simulink model "RL_UR3e_Pick_and_Place_Traj"  (R2024b)
settings: Solver=ode4  StartTime=0.0  StopTime=Tf  FixedStep=Ts_sim  RelTol=1e-3
values from neighbouring files (symbols this model uses):
  I_SCALE = 1 / I_max    (= 0.0104166666667)    [LQR_Gains.m]
  Ke = 0.0437    [LQR_Gains.m]
  Kt = 0.0437    [LQR_Gains.m]
  L = 0.001    [LQR_Gains.m]
  OMEGA_SCALE_J13 = 1 / pi    (= 0.318309886184)    [LQR_Gains.m]
  OMEGA_SCALE_J46 = 1 / (2*pi)    (= 0.159154943092)    [LQR_Gains.m]
  PICK = [-380, -170, 120]    [EvaluateAndAnalyzeAgents.m]    (also in Reward.m = PickTarget(:); TrainSACAgentForPickAndPlaceTraj.m; UR3eResetFcn.m; argetScheduler.m = Pick)
  PLACE = [-200,  -50, 300]    [EvaluateAndAnalyzeAgents.m]    (also in Reward.m = PlaceTarget(:); TrainSACAgentForPickAndPlaceTraj.m; UR3eResetFcn.m; argetScheduler.m = Place)
  R = 0.50    (= 0.5)    [LQR_Gains.m]
  Z_SCALE = Ts_sim    (= 0.005)    [LQR_Gains.m]
undefined symbols (not defined in the file or in its folder): b1, b2, b3, b4, b5, b6, InitTheta_1, InitTheta_2, InitTheta_3, InitTheta_4, InitTheta_5, InitTheta_6, J1, J2, J3, J4, J5, J6, K1, K2, K3, K4, K5, K6
libraries: rllib x1
(part 1 of 2)
settings Model: Creator=GigaByte Computers  LastModifiedBy=Acer
settings RTWCC: GPUComputeCapability=3.5

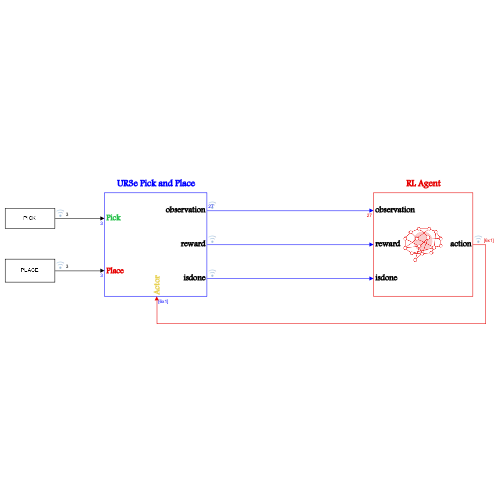
[thumbnail: Simulink's stored preview of the top-level diagram]
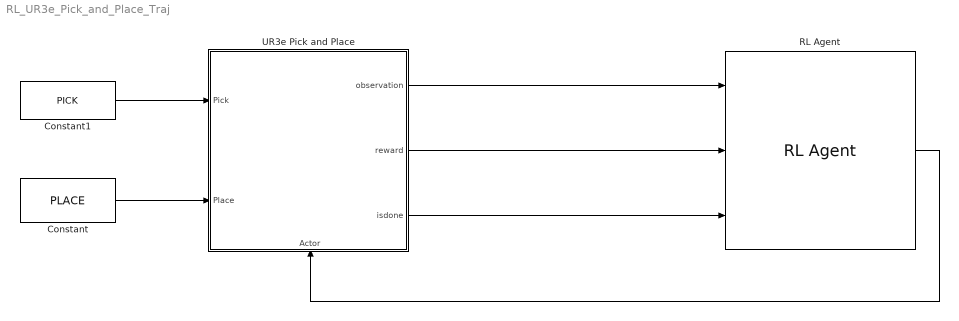
== system RL_UR3e_Pick_and_Place_Traj ==
  Constant : Constant  Value=PLACE
  Constant1 : Constant  Value=PICK
  RL Agent : rllib/RL Agent  Agent=agent  ExternalActionAsInput=off  ProvideLastAction=off  ProvideCumRwd=off  TreatAsDirectFeedthrough=on  UseStrictObservationDataTypes=off
  UR3e Pick and Place : Subsystem
      settings: PortSchema="{\"entries\":[{\"content\":{\"sides\":[{\"content\":{\"connectorIds\":[\"In1\",\"In2\"]},\"type\":\"ConnectorPlacement.EquallySpacedRectSide\",\"uuid\":\"13035aeb-c069-465b-bc28-233d93e7885c\"},{\"content\":{\"connectorIds\":[\"Out1\",\"Out2\",\"Out3\"],\"side\":\"RIGHT\"},\"type\":\"ConnectorPlacement.EquallySpacedRectSide\",\"uuid\":\"cbf2000c-b173-4779-ae30-0e5c1dcba60b\"},{\"content\":{\"connectorIds\":[\"In3\"],\"side\":\"TOP\"},\"type\":\"ConnectorPlacement.EquallySpacedRectSide\",\"uuid\":\"da0f4465-053c-4004-a8fa-0b8ae407464a\"}]},\"type\":\"ConnectorPlacement.EquallySpacedConnector\",\"uuid\":\"398c6cdf-546b-4a24-a522-29148214b593\"}],\"packageUris\":[\"http://schema.mathworks.com/mf0/Connector/R2020b\"],\"version\":\"1.0\"}"
  wires:
  UR3e Pick and Place/2(reward) -> RL Agent/2
  UR3e Pick and Place/1(isdone) -> RL Agent/3
  Constant/1 -> UR3e Pick and Place/1(Place)
  Constant1/1 -> UR3e Pick and Place/2(Pick)
  RL Agent/1 -> UR3e Pick and Place/3(Actor)
  UR3e Pick and Place/3(observation) -> RL Agent/1

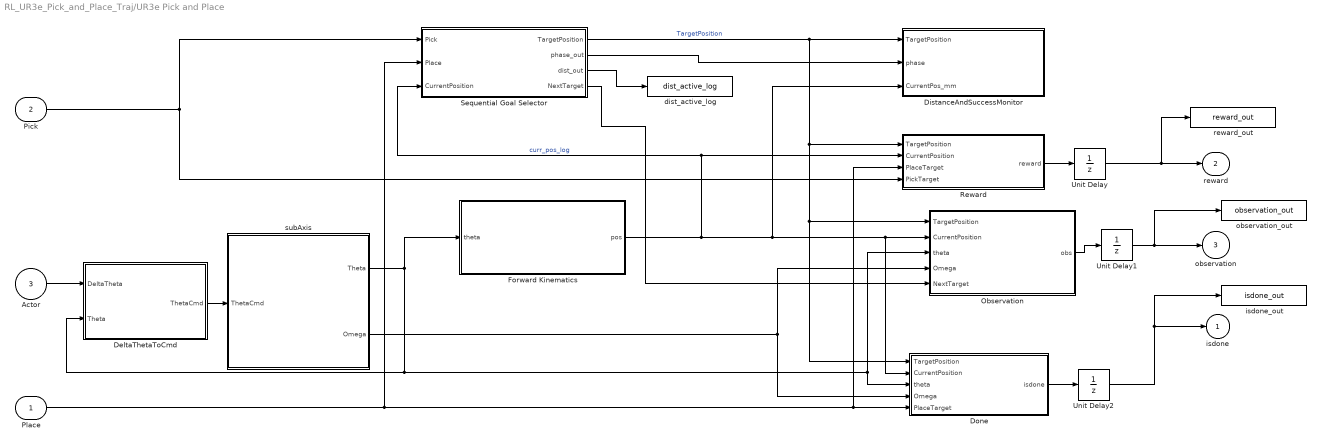
== system RL_UR3e_Pick_and_Place_Traj/UR3e Pick and Place ==
  Place : Inport
  Pick : Inport  Port=2
  Actor : Inport  Port=3
  DeltaThetaToCmd : MATLAB Function  TreatAsAtomicUnit=on
  DistanceAndSuccessMonitor : Subsystem
  Done : MATLAB Function
  Forward Kinematics : MATLAB Function
  Observation : MATLAB Function
  Reward : MATLAB Function
  Sequential Goal Selector : MATLAB Function  TreatAsAtomicUnit=on  SystemSampleTime=0.005
  Unit Delay : UnitDelay  SampleTime=-1  HasFrameUpgradeWarning=on
  Unit Delay1 : UnitDelay  SampleTime=-1  HasFrameUpgradeWarning=on
  Unit Delay2 : UnitDelay  InitialCondition=false  SampleTime=-1  HasFrameUpgradeWarning=on
  dist_active_log : ToWorkspace  VariableName=dist_active_log  SampleTime=-1
      settings: Save2DSignal=2-D array (concatenate along first dimension)
  isdone_out : ToWorkspace  VariableName=isdone_out  SampleTime=-1
      settings: Save2DSignal=2-D array (concatenate along first dimension)
  observation_out : ToWorkspace  VariableName=observation_out  SampleTime=-1
      settings: Save2DSignal=2-D array (concatenate along first dimension)
  reward_out : ToWorkspace  VariableName=reward_out  SampleTime=-1
      settings: Save2DSignal=2-D array (concatenate along first dimension)
  subAxis : Subsystem
  isdone : Outport
  reward : Outport  Port=2
  observation : Outport  Port=3
  wires:
  Reward/1(reward) -> Unit Delay/1
  Observation/1(obs) -> Unit Delay1/1
  Done/1(isdone) -> Unit Delay2/1
  Unit Delay/1 -> reward_out/1, reward/1
  Unit Delay1/1 -> observation_out/1, observation/1
  Unit Delay2/1 -> isdone_out/1, isdone/1
  subAxis/1(Theta) -> Forward Kinematics/1(theta), Observation/3(theta), Done/3(theta), DeltaThetaToCmd/2(Theta)
  subAxis/2(Omega) -> Observation/4(Omega), Done/4(Omega)
  Pick/1 -> Reward/4(PickTarget), Sequential Goal Selector/1(Pick)
  Place/1 -> Sequential Goal Selector/2(Place), Reward/3(PlaceTarget), Done/5(PlaceTarget)
  Sequential Goal Selector/1(TargetPosition) -> Reward/1(TargetPosition), Done/1(TargetPosition), Observation/1(TargetPosition), DistanceAndSuccessMonitor/1(TargetPosition)  "TargetPosition"
  Sequential Goal Selector/2(phase_out) -> DistanceAndSuccessMonitor/2(phase)
  Forward Kinematics/1(pos) -> Done/2(CurrentPosition), Observation/2(CurrentPosition), DistanceAndSuccessMonitor/3(CurrentPos_mm), Sequential Goal Selector/3(CurrentPosition), Reward/2(CurrentPosition)  "curr_pos_log"
  Sequential Goal Selector/3(dist_out) -> dist_active_log/1
  DeltaThetaToCmd/1(ThetaCmd) -> subAxis/1(ThetaCmd)
  Actor/1 -> DeltaThetaToCmd/1(DeltaTheta)
  Sequential Goal Selector/4(NextTarget) -> Observation/5(NextTarget)

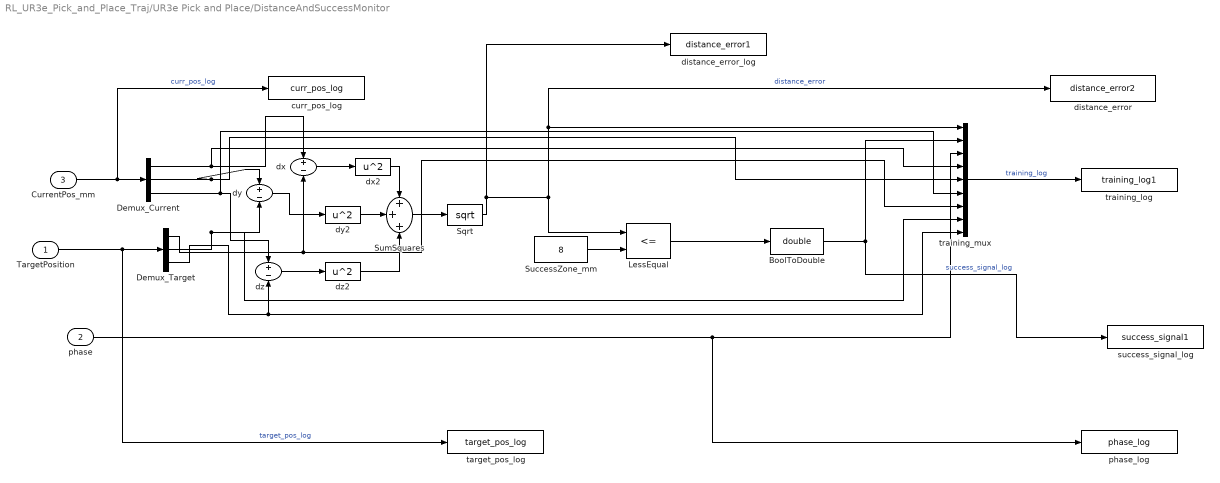
== system RL_UR3e_Pick_and_Place_Traj/UR3e Pick and Place/DistanceAndSuccessMonitor ==
  TargetPosition : Inport
  phase : Inport  Port=2
  CurrentPos_mm : Inport  Port=3
  BoolToDouble : DataTypeConversion  OutDataTypeStr=double  SaturateOnIntegerOverflow=off  RndMeth=Floor
  Demux_Current : Demux  Outputs=3
  Demux_Target : Demux  Outputs=3
  LessEqual : RelationalOperator  Operator=<=  OutDataTypeStr=boolean  RndMeth=Simplest  InputSameDT=off
  Sqrt : Math  Operator=sqrt
  SuccessZone_mm : Constant  Value=8
  SumSquares : Sum  Inputs=+++
  curr_pos_log : ToWorkspace  VariableName=curr_pos_log  SampleTime=-1
      settings: Save2DSignal=2-D array (concatenate along first dimension)
  distance_error : ToWorkspace  VariableName=distance_error2  SampleTime=-1
      settings: Save2DSignal=2-D array (concatenate along first dimension)
  distance_error_log : ToWorkspace  VariableName=distance_error1  SampleTime=-1
      settings: Save2DSignal=2-D array (concatenate along first dimension)
  dx : Sum  Inputs=+-
  dx2 : Math  Operator=square
  dy : Sum  Inputs=+-
  dy2 : Math  Operator=square
  dz : Sum  Inputs=+-
  dz2 : Math  Operator=square
  phase_log : ToWorkspace  VariableName=phase_log  SampleTime=-1
      settings: Save2DSignal=2-D array (concatenate along first dimension)
  success_signal_log : ToWorkspace  VariableName=success_signal1  SampleTime=-1
      settings: Save2DSignal=2-D array (concatenate along first dimension)
  target_pos_log : ToWorkspace  VariableName=target_pos_log  SampleTime=-1
      settings: Save2DSignal=2-D array (concatenate along first dimension)
  training_log : ToWorkspace  VariableName=training_log1  SampleTime=-1
      settings: Save2DSignal=2-D array (concatenate along first dimension)
  training_mux : Mux  Inputs=9
  wires:
  training_mux/1 -> training_log/1  "training_log"
  Demux_Target/1 -> dx/2, training_mux/7
  Demux_Target/3 -> dz/2, training_mux/9
  Demux_Current/2 -> dy/1, training_mux/5
  phase/1 -> phase_log/1, training_mux/3
  SuccessZone_mm/1 -> LessEqual/2
  Demux_Current/3 -> dz/1, training_mux/6
  dx2/1 -> SumSquares/1
  dy2/1 -> SumSquares/2
  dz2/1 -> SumSquares/3
  Sqrt/1 -> distance_error/1, training_mux/1, LessEqual/1, distance_error_log/1  "distance_error"
  SumSquares/1 -> Sqrt/1
  Demux_Target/2 -> dy/2, training_mux/8
  BoolToDouble/1 -> success_signal_log/1, training_mux/2  "success_signal_log"
  dy/1 -> dy2/1
  dz/1 -> dz2/1
  dx/1 -> dx2/1
  Demux_Current/1 -> dx/1, training_mux/4
  LessEqual/1 -> BoolToDouble/1
  TargetPosition/1 -> Demux_Target/1, target_pos_log/1  "target_pos_log"
  CurrentPos_mm/1 -> curr_pos_log/1, Demux_Current/1  "curr_pos_log"

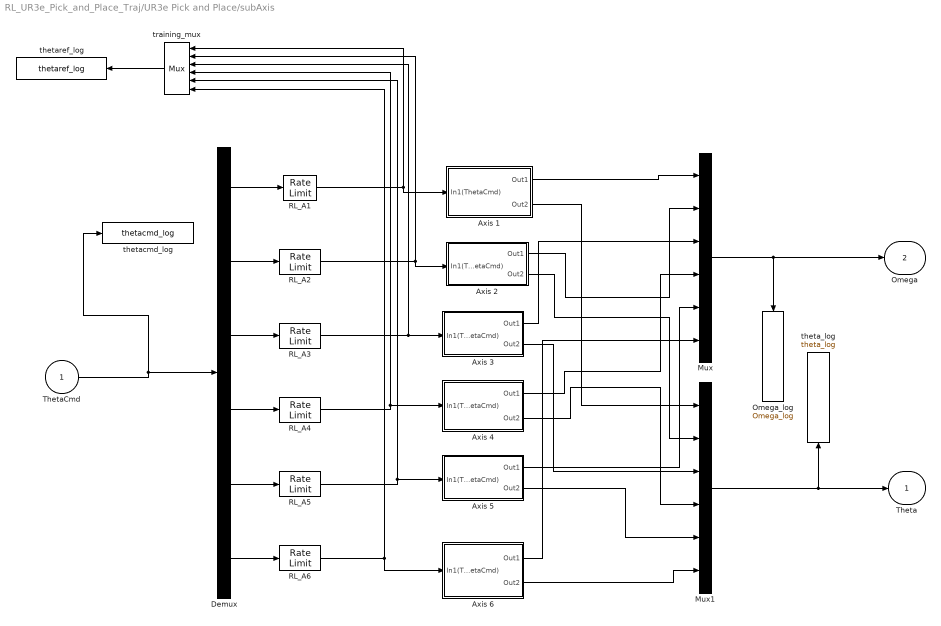
== system RL_UR3e_Pick_and_Place_Traj/UR3e Pick and Place/subAxis ==
  ThetaCmd : Inport
  Axis 1 : Subsystem
  Axis 2 : Subsystem
  Axis 3 : Subsystem
  Axis 4 : Subsystem
  Axis 5 : Subsystem
  Axis 6 : Subsystem
  Demux : Demux  Outputs=6
  Mux : Mux  Inputs=6
  Mux1 : Mux  Inputs=6
  Omega_log : ToWorkspace  VariableName=Omega_log  SampleTime=-1
      settings: Save2DSignal=2-D array (concatenate along first dimension)
  RL_A1 : RateLimiter  RisingSlewLimit=1*pi  FallingSlewLimit=-1*pi  SampleTimeMode=inherited
  RL_A2 : RateLimiter  RisingSlewLimit=1*pi  FallingSlewLimit=-1*pi  SampleTimeMode=inherited
  RL_A3 : RateLimiter  RisingSlewLimit=1*pi  FallingSlewLimit=-1*pi  SampleTimeMode=inherited
  RL_A4 : RateLimiter  RisingSlewLimit=2*pi  FallingSlewLimit=-2*pi  SampleTimeMode=inherited
  RL_A5 : RateLimiter  RisingSlewLimit=2*pi  FallingSlewLimit=-2*pi  SampleTimeMode=inherited
  RL_A6 : RateLimiter  RisingSlewLimit=2*pi  FallingSlewLimit=-2*pi  SampleTimeMode=inherited
  theta_log : ToWorkspace  VariableName=theta_log  SampleTime=-1
      settings: Save2DSignal=2-D array (concatenate along first dimension)
  thetacmd_log : ToWorkspace  VariableName=thetacmd_log  SampleTime=-1
      settings: Save2DSignal=2-D array (concatenate along first dimension)
  thetaref_log : ToWorkspace  VariableName=thetaref_log  SampleTime=-1
      settings: Save2DSignal=2-D array (concatenate along first dimension)
  training_mux : Mux  Inputs=6
  Theta : Outport
  Omega : Outport  Port=2
  wires:
  Demux/5 -> RL_A5/1
  Axis 5/1(Out1) -> Mux/5
  Axis 6/1(Out1) -> Mux/6
  Axis 2/2(Out2) -> Mux1/2
  Axis 3/2(Out2) -> Mux1/3
  Axis 5/2(Out2) -> Mux1/5
  Axis 2/1(Out1) -> Mux/2
  Demux/2 -> RL_A2/1
  Demux/3 -> RL_A3/1
  Axis 4/2(Out2) -> Mux1/4
  Demux/1 -> RL_A1/1
  Axis 1/1(Out1) -> Mux/1
  Axis 1/2(Out2) -> Mux1/1
  Axis 4/1(Out1) -> Mux/4
  Demux/4 -> RL_A4/1
  Axis 6/2(Out2) -> Mux1/6
  Demux/6 -> RL_A6/1
  Axis 3/1(Out1) -> Mux/3
  Mux1/1 -> Theta/1, theta_log/1
  ThetaCmd/1 -> Demux/1, thetacmd_log/1
  Mux/1 -> Omega_log/1, Omega/1
  RL_A1/1 -> Axis 1/1(In1(ThetaCmd)), training_mux/1
  RL_A6/1 -> Axis 6/1(In1(ThetaCmd)), training_mux/6
  RL_A2/1 -> Axis 2/1(In1(ThetaCmd)), training_mux/2
  RL_A3/1 -> training_mux/3, Axis 3/1(In1(ThetaCmd))
  RL_A4/1 -> Axis 4/1(In1(ThetaCmd)), training_mux/4
  RL_A5/1 -> Axis 5/1(In1(ThetaCmd)), training_mux/5
  training_mux/1 -> thetaref_log/1

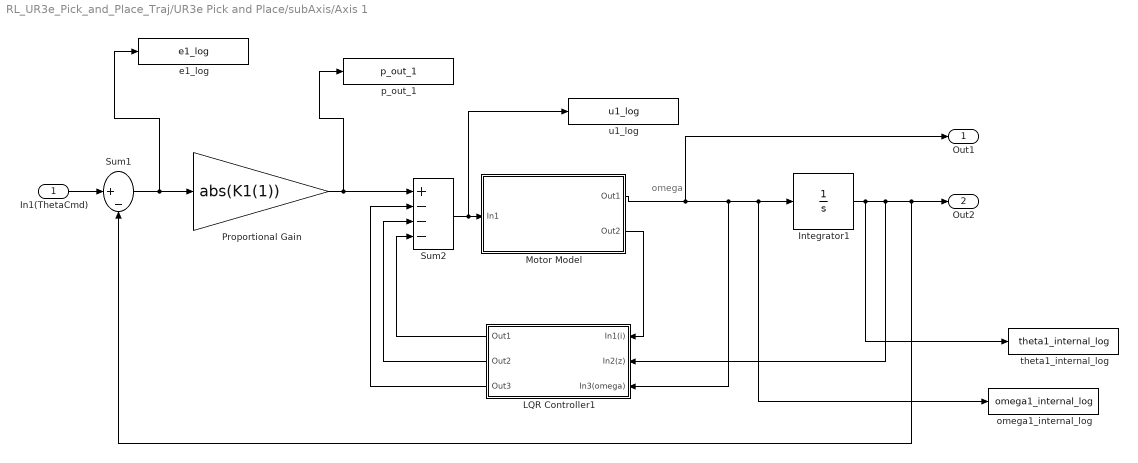
== system RL_UR3e_Pick_and_Place_Traj/UR3e Pick and Place/subAxis/Axis 1 ==
  note: omega
  In1(ThetaCmd) : Inport
  Integrator1 : Integrator  InitialCondition=InitTheta_1
  LQR Controller1 : Subsystem
  Motor Model : Subsystem
  Proportional Gain : Gain  Gain=abs(K1(1))
  Sum1 : Sum  Inputs=|+-
  Sum2 : Sum  Inputs=+---
  e1_log : ToWorkspace  VariableName=e1_log  SampleTime=-1
      settings: Save2DSignal=2-D array (concatenate along first dimension)
  omega1_internal_log : ToWorkspace  VariableName=omega1_internal_log  SampleTime=-1
      settings: Save2DSignal=2-D array (concatenate along first dimension)
  p_out_1 : ToWorkspace  VariableName=p_out_1  SampleTime=-1
      settings: Save2DSignal=2-D array (concatenate along first dimension)
  theta1_internal_log : ToWorkspace  VariableName=theta1_internal_log  SampleTime=-1
      settings: Save2DSignal=2-D array (concatenate along first dimension)
  u1_log : ToWorkspace  VariableName=u1_log  SampleTime=-1
      settings: Save2DSignal=2-D array (concatenate along first dimension)
  Out1 : Outport
  Out2 : Outport  Port=2
  wires:
  Sum2/1 -> u1_log/1, Motor Model/1(In1)
  Motor Model/1(Out1) -> Out1/1, LQR Controller1/3(In3(omega)), omega1_internal_log/1, Integrator1/1
  Sum1/1 -> e1_log/1, Proportional Gain/1
  Proportional Gain/1 -> p_out_1/1, Sum2/1
  In1(ThetaCmd)/1 -> Sum1/1
  LQR Controller1/1(Out1) -> Sum2/4
  LQR Controller1/2(Out2) -> Sum2/3
  LQR Controller1/3(Out3) -> Sum2/2
  Integrator1/1 -> theta1_internal_log/1, LQR Controller1/2("In2(z) "), Sum1/2, Out2/1
  Motor Model/2(Out2) -> LQR Controller1/1("In1(i) ")

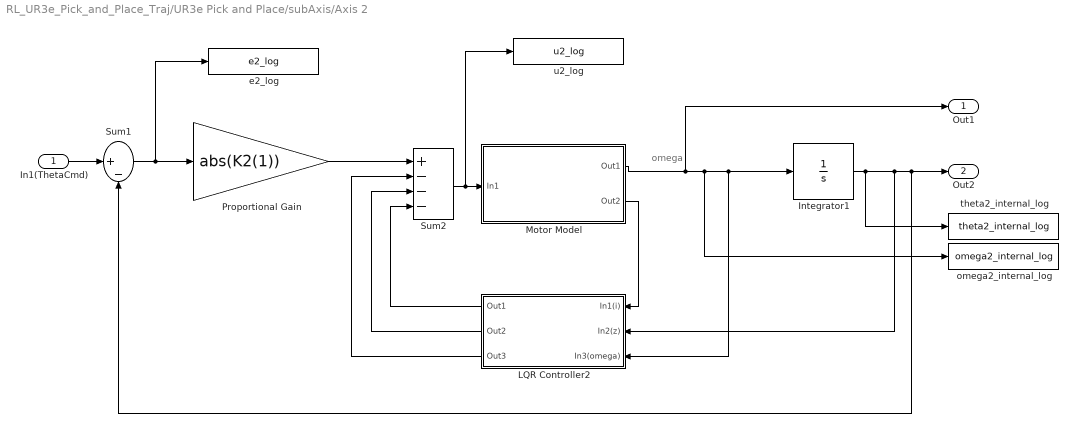
== system RL_UR3e_Pick_and_Place_Traj/UR3e Pick and Place/subAxis/Axis 2 ==
  note: omega
  In1(ThetaCmd) : Inport
  Integrator1 : Integrator  InitialCondition=InitTheta_2
  LQR Controller2 : Subsystem
  Motor Model : Subsystem
  Proportional Gain : Gain  Gain=abs(K2(1))
  Sum1 : Sum  Inputs=|+-
  Sum2 : Sum  Inputs=+---
  e2_log : ToWorkspace  VariableName=e2_log  SampleTime=-1
      settings: Save2DSignal=2-D array (concatenate along first dimension)
  omega2_internal_log : ToWorkspace  VariableName=omega2_internal_log  SampleTime=-1
      settings: Save2DSignal=2-D array (concatenate along first dimension)
  theta2_internal_log : ToWorkspace  VariableName=theta2_internal_log  SampleTime=-1
      settings: Save2DSignal=2-D array (concatenate along first dimension)
  u2_log : ToWorkspace  VariableName=u2_log  SampleTime=-1
      settings: Save2DSignal=2-D array (concatenate along first dimension)
  Out1 : Outport
  Out2 : Outport  Port=2
  wires:
  Proportional Gain/1 -> Sum2/1
  Motor Model/1(Out1) -> Out1/1, omega2_internal_log/1, LQR Controller2/3(In3(omega)), Integrator1/1
  LQR Controller2/2(Out2) -> Sum2/3
  Motor Model/2(Out2) -> LQR Controller2/1("In1(i) ")
  In1(ThetaCmd)/1 -> Sum1/1
  LQR Controller2/3(Out3) -> Sum2/2
  LQR Controller2/1(Out1) -> Sum2/4
  Sum1/1 -> e2_log/1, Proportional Gain/1
  Integrator1/1 -> theta2_internal_log/1, LQR Controller2/2("In2(z) "), Sum1/2, Out2/1
  Sum2/1 -> u2_log/1, Motor Model/1(In1)

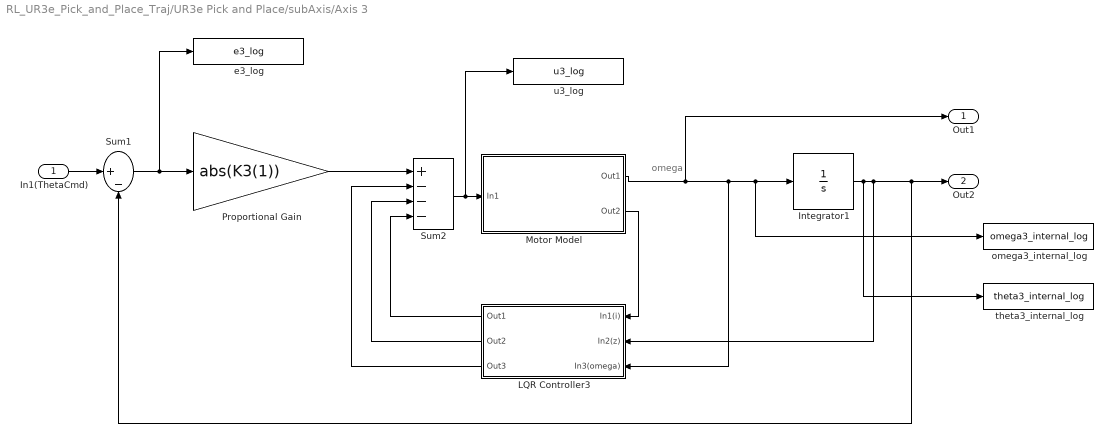
== system RL_UR3e_Pick_and_Place_Traj/UR3e Pick and Place/subAxis/Axis 3 ==
  note: omega
  In1(ThetaCmd) : Inport
  Integrator1 : Integrator  InitialCondition=InitTheta_3
  LQR Controller3 : Subsystem
  Motor Model : Subsystem
  Proportional Gain : Gain  Gain=abs(K3(1))
  Sum1 : Sum  Inputs=|+-
  Sum2 : Sum  Inputs=+---
  e3_log : ToWorkspace  VariableName=e3_log  SampleTime=-1
      settings: Save2DSignal=2-D array (concatenate along first dimension)
  omega3_internal_log : ToWorkspace  VariableName=omega3_internal_log  SampleTime=-1
      settings: Save2DSignal=2-D array (concatenate along first dimension)
  theta3_internal_log : ToWorkspace  VariableName=theta3_internal_log  SampleTime=-1
      settings: Save2DSignal=2-D array (concatenate along first dimension)
  u3_log : ToWorkspace  VariableName=u3_log  SampleTime=-1
      settings: Save2DSignal=2-D array (concatenate along first dimension)
  Out1 : Outport
  Out2 : Outport  Port=2
  wires:
  Sum2/1 -> u3_log/1, Motor Model/1(In1)
  Integrator1/1 -> theta3_internal_log/1, LQR Controller3/2("In2(z) "), Sum1/2, Out2/1
  Sum1/1 -> e3_log/1, Proportional Gain/1
  LQR Controller3/3(Out3) -> Sum2/2
  LQR Controller3/1(Out1) -> Sum2/4
  In1(ThetaCmd)/1 -> Sum1/1
  Motor Model/2(Out2) -> LQR Controller3/1("In1(i) ")
  Motor Model/1(Out1) -> Out1/1, omega3_internal_log/1, Integrator1/1, LQR Controller3/3(In3(omega))
  Proportional Gain/1 -> Sum2/1
  LQR Controller3/2(Out2) -> Sum2/3

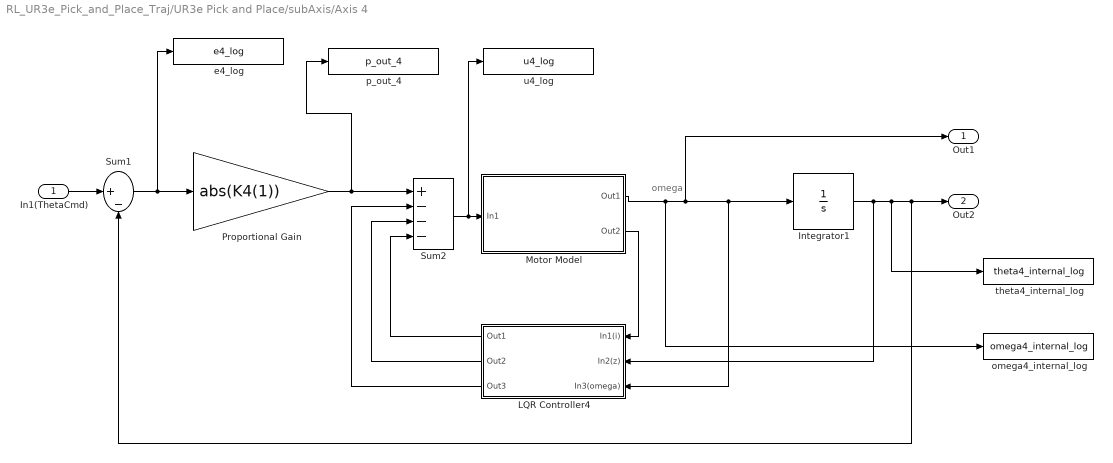
== system RL_UR3e_Pick_and_Place_Traj/UR3e Pick and Place/subAxis/Axis 4 ==
  note: omega
  In1(ThetaCmd) : Inport
  Integrator1 : Integrator  InitialCondition=InitTheta_4
  LQR Controller4 : Subsystem
  Motor Model : Subsystem
  Proportional Gain : Gain  Gain=abs(K4(1))
  Sum1 : Sum  Inputs=|+-
  Sum2 : Sum  Inputs=+---
  e4_log : ToWorkspace  VariableName=e4_log  SampleTime=-1
      settings: Save2DSignal=2-D array (concatenate along first dimension)
  omega4_internal_log : ToWorkspace  VariableName=omega4_internal_log  SampleTime=-1
      settings: Save2DSignal=2-D array (concatenate along first dimension)
  p_out_4 : ToWorkspace  VariableName=p_out_4  SampleTime=-1
      settings: Save2DSignal=2-D array (concatenate along first dimension)
  theta4_internal_log : ToWorkspace  VariableName=theta4_internal_log  SampleTime=-1
      settings: Save2DSignal=2-D array (concatenate along first dimension)
  u4_log : ToWorkspace  VariableName=u4_log  SampleTime=-1
      settings: Save2DSignal=2-D array (concatenate along first dimension)
  Out1 : Outport
  Out2 : Outport  Port=2
  wires:
  LQR Controller4/2(Out2) -> Sum2/3
  Proportional Gain/1 -> p_out_4/1, Sum2/1
  LQR Controller4/3(Out3) -> Sum2/2
  Sum1/1 -> e4_log/1, Proportional Gain/1
  Integrator1/1 -> LQR Controller4/2("In2(z) "), theta4_internal_log/1, Sum1/2, Out2/1
  Motor Model/1(Out1) -> omega4_internal_log/1, Out1/1, LQR Controller4/3(In3(omega)), Integrator1/1
  Motor Model/2(Out2) -> LQR Controller4/1("In1(i) ")
  LQR Controller4/1(Out1) -> Sum2/4
  In1(ThetaCmd)/1 -> Sum1/1
  Sum2/1 -> u4_log/1, Motor Model/1(In1)

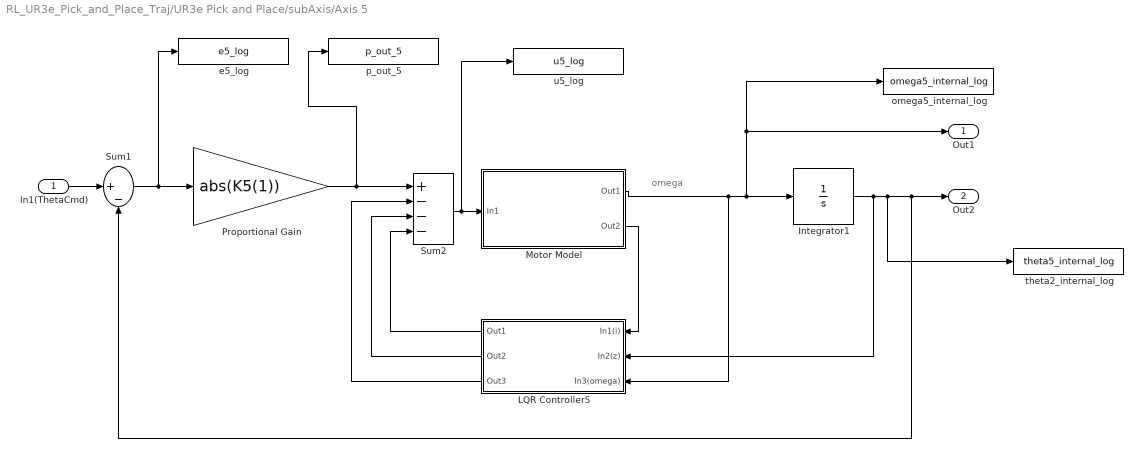
== system RL_UR3e_Pick_and_Place_Traj/UR3e Pick and Place/subAxis/Axis 5 ==
  note: omega
  In1(ThetaCmd) : Inport
  Integrator1 : Integrator  InitialCondition=InitTheta_5
  LQR Controller5 : Subsystem
  Motor Model : Subsystem
  Proportional Gain : Gain  Gain=abs(K5(1))
  Sum1 : Sum  Inputs=|+-
  Sum2 : Sum  Inputs=+---
  e5_log : ToWorkspace  VariableName=e5_log  SampleTime=-1
      settings: Save2DSignal=2-D array (concatenate along first dimension)
  omega5_internal_log : ToWorkspace  VariableName=omega5_internal_log  SampleTime=-1
      settings: Save2DSignal=2-D array (concatenate along first dimension)
  p_out_5 : ToWorkspace  VariableName=p_out_5  SampleTime=-1
      settings: Save2DSignal=2-D array (concatenate along first dimension)
  theta2_internal_log : ToWorkspace  VariableName=theta5_internal_log  SampleTime=-1
      settings: Save2DSignal=2-D array (concatenate along first dimension)
  u5_log : ToWorkspace  VariableName=u5_log  SampleTime=-1
      settings: Save2DSignal=2-D array (concatenate along first dimension)
  Out1 : Outport
  Out2 : Outport  Port=2
  wires:
  Proportional Gain/1 -> p_out_5/1, Sum2/1
  LQR Controller5/2(Out2) -> Sum2/3
  Sum2/1 -> u5_log/1, Motor Model/1(In1)
  Motor Model/2(Out2) -> LQR Controller5/1("In1(i) ")
  LQR Controller5/1(Out1) -> Sum2/4
  Motor Model/1(Out1) -> omega5_internal_log/1, Out1/1, Integrator1/1, LQR Controller5/3(In3(omega))
  In1(ThetaCmd)/1 -> Sum1/1
  Sum1/1 -> e5_log/1, Proportional Gain/1
  Integrator1/1 -> LQR Controller5/2("In2(z) "), theta2_internal_log/1, Sum1/2, Out2/1
  LQR Controller5/3(Out3) -> Sum2/2

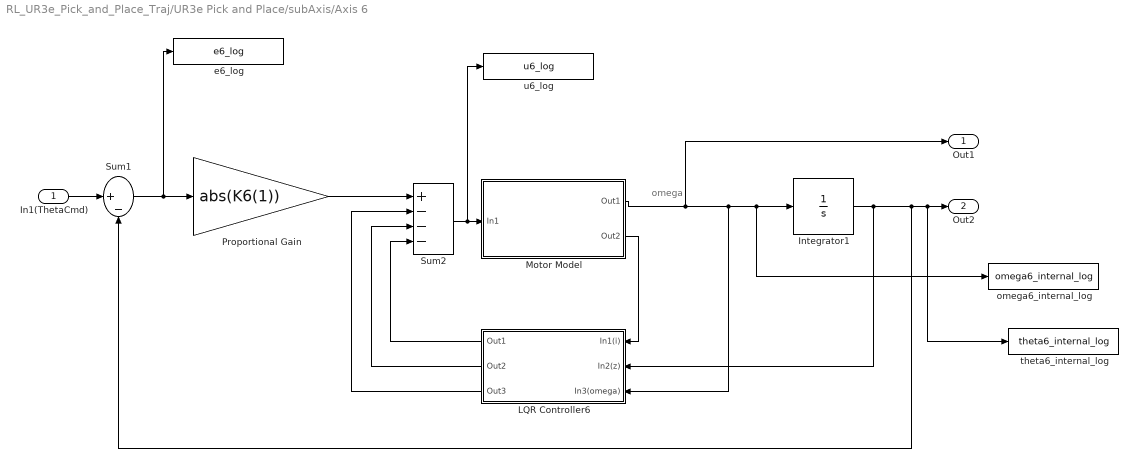
== system RL_UR3e_Pick_and_Place_Traj/UR3e Pick and Place/subAxis/Axis 6 ==
  note: omega
  In1(ThetaCmd) : Inport
  Integrator1 : Integrator  InitialCondition=InitTheta_6
  LQR Controller6 : Subsystem
  Motor Model : Subsystem
  Proportional Gain : Gain  Gain=abs(K6(1))
  Sum1 : Sum  Inputs=|+-
  Sum2 : Sum  Inputs=+---
  e6_log : ToWorkspace  VariableName=e6_log  SampleTime=-1
      settings: Save2DSignal=2-D array (concatenate along first dimension)
  omega6_internal_log : ToWorkspace  VariableName=omega6_internal_log  SampleTime=-1
      settings: Save2DSignal=2-D array (concatenate along first dimension)
  theta6_internal_log : ToWorkspace  VariableName=theta6_internal_log  SampleTime=-1
      settings: Save2DSignal=2-D array (concatenate along first dimension)
  u6_log : ToWorkspace  VariableName=u6_log  SampleTime=-1
      settings: Save2DSignal=2-D array (concatenate along first dimension)
  Out1 : Outport
  Out2 : Outport  Port=2
  wires:
  LQR Controller6/1(Out1) -> Sum2/4
  LQR Controller6/2(Out2) -> Sum2/3
  Motor Model/2(Out2) -> LQR Controller6/1("In1(i) ")
  Proportional Gain/1 -> Sum2/1
  Integrator1/1 -> LQR Controller6/2("In2(z) "), Sum1/2, theta6_internal_log/1, Out2/1
  Sum2/1 -> u6_log/1, Motor Model/1(In1)
  LQR Controller6/3(Out3) -> Sum2/2
  Motor Model/1(Out1) -> Out1/1, LQR Controller6/3(In3(omega)), omega6_internal_log/1, Integrator1/1
  Sum1/1 -> e6_log/1, Proportional Gain/1
  In1(ThetaCmd)/1 -> Sum1/1

== system RL_UR3e_Pick_and_Place_Traj/UR3e Pick and Place/subAxis/Axis 1/LQR Controller1 ==
  "In1(i) " : Inport
  "In2(z) " : Inport  Port=2
  In3(omega) : Inport  Port=3
  Gain omega : Gain  Gain=K1(3)*OMEGA_SCALE_J13
  Gain_i : Gain  Gain=K1(4)*I_SCALE
  Gain_z : Gain  Gain=K1(2)*Z_SCALE
  Out1 : Outport
  Out2 : Outport  Port=2
  Out3 : Outport  Port=3
  wires:
  "In2(z) "/1 -> Gain_z/1
  Gain_i/1 -> Out1/1
  "In1(i) "/1 -> Gain_i/1
  Gain omega/1 -> Out3/1
  Gain_z/1 -> Out2/1
  In3(omega)/1 -> Gain omega/1

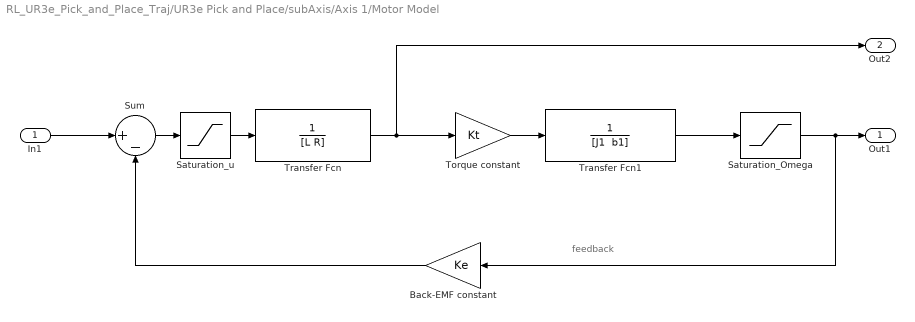
== system RL_UR3e_Pick_and_Place_Traj/UR3e Pick and Place/subAxis/Axis 1/Motor Model ==
  note: feedback
  In1 : Inport
  Back-EMF constant : Gain  Gain=Ke
  Saturation_Omega : Saturate  UpperLimit=1*pi  LowerLimit=-1*pi
  Saturation_u : Saturate  UpperLimit=48  LowerLimit=-48
  Sum : Sum  Inputs=|+-
  Torque constant : Gain  Gain=Kt
  Transfer Fcn : TransferFcn  Denominator=[L R]
  Transfer Fcn1 : TransferFcn  Denominator="[J1  b1]"
  Out1 : Outport
  Out2 : Outport  Port=2
  wires:
  In1/1 -> Sum/1
  Transfer Fcn/1 -> Torque constant/1, Out2/1
  Back-EMF constant/1 -> Sum/2
  Transfer Fcn1/1 -> Saturation_Omega/1
  Torque constant/1 -> Transfer Fcn1/1
  Sum/1 -> Saturation_u/1
  Saturation_u/1 -> Transfer Fcn/1
  Saturation_Omega/1 -> Back-EMF constant/1, Out1/1

== system RL_UR3e_Pick_and_Place_Traj/UR3e Pick and Place/subAxis/Axis 2/LQR Controller2 ==
  "In1(i) " : Inport
  "In2(z) " : Inport  Port=2
  In3(omega) : Inport  Port=3
  Gain omega : Gain  Gain=K2(3)*OMEGA_SCALE_J13
  Gain_i : Gain  Gain=K2(4)*I_SCALE
  Gain_z : Gain  Gain=K2(2)*Z_SCALE
  Out1 : Outport
  Out2 : Outport  Port=2
  Out3 : Outport  Port=3
  wires:
  "In2(z) "/1 -> Gain_z/1
  Gain_i/1 -> Out1/1
  "In1(i) "/1 -> Gain_i/1
  Gain omega/1 -> Out3/1
  Gain_z/1 -> Out2/1
  In3(omega)/1 -> Gain omega/1

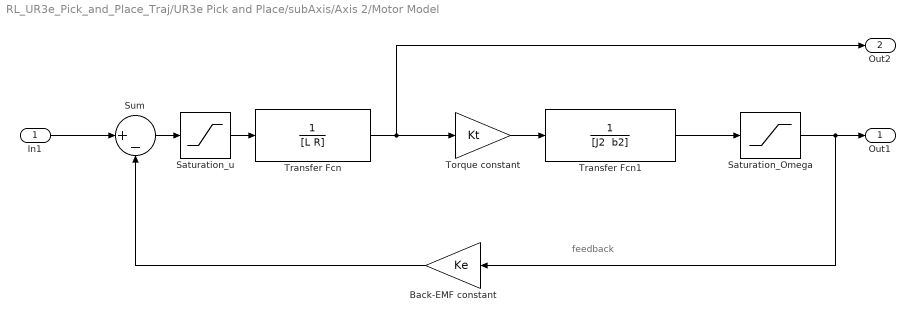
== system RL_UR3e_Pick_and_Place_Traj/UR3e Pick and Place/subAxis/Axis 2/Motor Model ==
  note: feedback
  In1 : Inport
  Back-EMF constant : Gain  Gain=Ke
  Saturation_Omega : Saturate  UpperLimit=1*pi  LowerLimit=-1*pi
  Saturation_u : Saturate  UpperLimit=48  LowerLimit=-48
  Sum : Sum  Inputs=|+-
  Torque constant : Gain  Gain=Kt
  Transfer Fcn : TransferFcn  Denominator=[L R]
  Transfer Fcn1 : TransferFcn  Denominator="[J2  b2]"
  Out1 : Outport
  Out2 : Outport  Port=2
  wires:
  In1/1 -> Sum/1
  Transfer Fcn/1 -> Torque constant/1, Out2/1
  Back-EMF constant/1 -> Sum/2
  Transfer Fcn1/1 -> Saturation_Omega/1
  Torque constant/1 -> Transfer Fcn1/1
  Sum/1 -> Saturation_u/1
  Saturation_u/1 -> Transfer Fcn/1
  Saturation_Omega/1 -> Back-EMF constant/1, Out1/1

== system RL_UR3e_Pick_and_Place_Traj/UR3e Pick and Place/subAxis/Axis 3/LQR Controller3 ==
  "In1(i) " : Inport
  "In2(z) " : Inport  Port=2
  In3(omega) : Inport  Port=3
  Gain omega : Gain  Gain=K3(3)*OMEGA_SCALE_J13
  Gain_i : Gain  Gain=K3(4)*I_SCALE
  Gain_z : Gain  Gain=K3(2)*Z_SCALE
  Out1 : Outport
  Out2 : Outport  Port=2
  Out3 : Outport  Port=3
  wires:
  "In2(z) "/1 -> Gain_z/1
  Gain_i/1 -> Out1/1
  "In1(i) "/1 -> Gain_i/1
  Gain omega/1 -> Out3/1
  Gain_z/1 -> Out2/1
  In3(omega)/1 -> Gain omega/1

== system RL_UR3e_Pick_and_Place_Traj/UR3e Pick and Place/subAxis/Axis 3/Motor Model ==
  note: feedback
  In1 : Inport
  Back-EMF constant : Gain  Gain=Ke
  Saturation_Omega : Saturate  UpperLimit=1*pi  LowerLimit=-1*pi
  Saturation_u : Saturate  UpperLimit=48  LowerLimit=-48
  Sum : Sum  Inputs=|+-
  Torque constant : Gain  Gain=Kt
  Transfer Fcn : TransferFcn  Denominator=[L R]
  Transfer Fcn1 : TransferFcn  Denominator="[J3  b3]"
  Out1 : Outport
  Out2 : Outport  Port=2
  wires:
  In1/1 -> Sum/1
  Transfer Fcn/1 -> Torque constant/1, Out2/1
  Back-EMF constant/1 -> Sum/2
  Transfer Fcn1/1 -> Saturation_Omega/1
  Torque constant/1 -> Transfer Fcn1/1
  Sum/1 -> Saturation_u/1
  Saturation_u/1 -> Transfer Fcn/1
  Saturation_Omega/1 -> Back-EMF constant/1, Out1/1

== system RL_UR3e_Pick_and_Place_Traj/UR3e Pick and Place/subAxis/Axis 4/LQR Controller4 ==
  "In1(i) " : Inport
  "In2(z) " : Inport  Port=2
  In3(omega) : Inport  Port=3
  Gain omega : Gain  Gain=K4(3)*OMEGA_SCALE_J46
  Gain_i : Gain  Gain=K4(4)*I_SCALE
  Gain_z : Gain  Gain=K4(2)*Z_SCALE
  Out1 : Outport
  Out2 : Outport  Port=2
  Out3 : Outport  Port=3
  wires:
  "In2(z) "/1 -> Gain_z/1
  Gain_i/1 -> Out1/1
  "In1(i) "/1 -> Gain_i/1
  Gain omega/1 -> Out3/1
  Gain_z/1 -> Out2/1
  In3(omega)/1 -> Gain omega/1

== system RL_UR3e_Pick_and_Place_Traj/UR3e Pick and Place/subAxis/Axis 4/Motor Model ==
  note: feedback
  In1 : Inport
  Back-EMF constant : Gain  Gain=Ke
  Saturation_Omega : Saturate  UpperLimit=2*pi  LowerLimit=-2*pi
  Saturation_u : Saturate  UpperLimit=48  LowerLimit=-48
  Sum : Sum  Inputs=|+-
  Torque constant : Gain  Gain=Kt
  Transfer Fcn : TransferFcn  Denominator=[L R]
  Transfer Fcn1 : TransferFcn  Denominator="[J4  b4]"
  Out1 : Outport
  Out2 : Outport  Port=2
  wires:
  In1/1 -> Sum/1
  Transfer Fcn/1 -> Torque constant/1, Out2/1
  Back-EMF constant/1 -> Sum/2
  Transfer Fcn1/1 -> Saturation_Omega/1
  Torque constant/1 -> Transfer Fcn1/1
  Sum/1 -> Saturation_u/1
  Saturation_u/1 -> Transfer Fcn/1
  Saturation_Omega/1 -> Back-EMF constant/1, Out1/1

== system RL_UR3e_Pick_and_Place_Traj/UR3e Pick and Place/subAxis/Axis 5/LQR Controller5 ==
  "In1(i) " : Inport
  "In2(z) " : Inport  Port=2
  In3(omega) : Inport  Port=3
  Gain omega : Gain  Gain=K5(3)*OMEGA_SCALE_J46
  Gain_i : Gain  Gain=K5(4)*I_SCALE
  Gain_z : Gain  Gain=K5(2)*Z_SCALE
  Out1 : Outport
  Out2 : Outport  Port=2
  Out3 : Outport  Port=3
  wires:
  "In2(z) "/1 -> Gain_z/1
  Gain_i/1 -> Out1/1
  "In1(i) "/1 -> Gain_i/1
  Gain omega/1 -> Out3/1
  Gain_z/1 -> Out2/1
  In3(omega)/1 -> Gain omega/1

== system RL_UR3e_Pick_and_Place_Traj/UR3e Pick and Place/subAxis/Axis 5/Motor Model ==
  note: feedback
  In1 : Inport
  Back-EMF constant : Gain  Gain=Ke
  Saturation_Omega : Saturate  UpperLimit=2*pi  LowerLimit=-2*pi
  Saturation_u : Saturate  UpperLimit=48  LowerLimit=-48
  Sum : Sum  Inputs=|+-
  Torque constant : Gain  Gain=Kt
  Transfer Fcn : TransferFcn  Denominator=[L R]
  Transfer Fcn1 : TransferFcn  Denominator="[J5  b5]"
  Out1 : Outport
  Out2 : Outport  Port=2
  wires:
  In1/1 -> Sum/1
  Transfer Fcn/1 -> Torque constant/1, Out2/1
  Back-EMF constant/1 -> Sum/2
  Transfer Fcn1/1 -> Saturation_Omega/1
  Torque constant/1 -> Transfer Fcn1/1
  Sum/1 -> Saturation_u/1
  Saturation_u/1 -> Transfer Fcn/1
  Saturation_Omega/1 -> Back-EMF constant/1, Out1/1

== system RL_UR3e_Pick_and_Place_Traj/UR3e Pick and Place/subAxis/Axis 6/LQR Controller6 ==
  "In1(i) " : Inport
  "In2(z) " : Inport  Port=2
  In3(omega) : Inport  Port=3
  Gain omega : Gain  Gain=K6(3)*OMEGA_SCALE_J46
  Gain_i : Gain  Gain=K6(4)*I_SCALE
  Gain_z : Gain  Gain=K6(2)*Z_SCALE
  Out1 : Outport
  Out2 : Outport  Port=2
  Out3 : Outport  Port=3
  wires:
  "In2(z) "/1 -> Gain_z/1
  Gain_i/1 -> Out1/1
  "In1(i) "/1 -> Gain_i/1
  Gain omega/1 -> Out3/1
  Gain_z/1 -> Out2/1
  In3(omega)/1 -> Gain omega/1

== system RL_UR3e_Pick_and_Place_Traj/UR3e Pick and Place/subAxis/Axis 6/Motor Model ==
  note: feedback
  In1 : Inport
  Back-EMF constant : Gain  Gain=Ke
  Saturation_Omega : Saturate  UpperLimit=2*pi  LowerLimit=-2*pi
  Saturation_u : Saturate  UpperLimit=48  LowerLimit=-48
  Sum : Sum  Inputs=|+-
  Torque constant : Gain  Gain=Kt
  Transfer Fcn : TransferFcn  Denominator=[L R]
  Transfer Fcn1 : TransferFcn  Denominator="[J6  b6]"
  Out1 : Outport
  Out2 : Outport  Port=2
  wires:
  In1/1 -> Sum/1
  Transfer Fcn/1 -> Torque constant/1, Out2/1
  Back-EMF constant/1 -> Sum/2
  Transfer Fcn1/1 -> Saturation_Omega/1
  Torque constant/1 -> Transfer Fcn1/1
  Sum/1 -> Saturation_u/1
  Saturation_u/1 -> Transfer Fcn/1
  Saturation_Omega/1 -> Back-EMF constant/1, Out1/1

== matlab function RL_UR3e_Pick_and_Place_Traj/UR3e Pick and Place/Reward ==
  settings: updateMethod=DISCRETE
  data: TargetPosition input; CurrentPosition input; PlaceTarget input; reward output; PickTarget input
function reward = Reward(TargetPosition, CurrentPosition, PlaceTarget, PickTarget)
%% =========================================================================
%  FILE     : Reward.m
%  PROJECT  : UR3e Reinforcement Learning Framework — Project #1
%  VERSION  : v19.7
%  DATE     : 24-Apr-2026
%
%  AUTHOR   : Ahmed Iqdymat
%  AFFIL.   : University Politehnica of Bucharest
%  SUPERV.  : Dr. Grigore Stamatescu
%
%  FUNCTION SIGNATURE: UNCHANGED (same 4 inputs as v15.2 / v19.4)
%
%  EVIDENCE-BASED RATIONALE FOR v19.7
%  -------------------------------------------------------------------------
%  Four prior evaluations on the same environment (same Observation,
%  Done, TargetScheduler and ResetFcn blocks) converged on a single
%  structural conclusion: the intermediate-waypoint reward is already
%  correct, and the remaining task-completion gap lives entirely in the
%  terminal waypoints.
%
%    V1 (v19.4, 1000 ep): PickRate = LiftRate = CruiseRate = 100 %,
%        MinCruise = 40.84 mm, MaxPhase = 3. Intermediate policy
%        stable; CRUISE barrier prevented Phase 4 entry.
%
%    V2 (v19.5, 2000 ep): graded ramp plus 80 mm approach zone for
%        every waypoint. LiftRate dropped to 0 %, MinPick = 32.27 mm.
%        Outer slope −1.82 /mm and inner slope −20 /mm produced a
%        non-convex landscape with a reward-farming region.
%
%    V2.1 (v19.6, ~1400 ep): intermediate threshold widened 25 → 40 mm.
%         Average reward collapsed to 2.42, Q0 drifted to −10.8. The
%         policy learned net-backward motion.
%
%    V1 retry (v19.4, 5000 ep): Phase 4 now entered in 20/20 episodes,
%        MinPlace improved from 152 mm (V1) to 26.24 mm, but remained
%        outside the 8 mm tolerance (PlaceZone8mm = 0 %). MinCruise
%        converged to 25.04 ± 0.03 mm — an extreme edge-hovering
%        signature at exactly the TargetScheduler threshold. MinPlace
%        exhibited a different pattern: 26.24 ± 3.94 mm, σ/tol ≈ 49 %,
%        i.e. the policy did not find a stable attractor inside the
%        8 mm PLACE tolerance and instead stopped wherever the local
%        progress reward ceased to improve.
%
%  DIAGNOSIS
%  -------------------------------------------------------------------------
%  The flat +500 bonus in v19.4 creates a reward plateau inside each
%  tolerance with no internal gradient (∂R/∂d = 0 for d < tol) and a
%  step discontinuity at d = tol. For the 25 mm intermediate tolerances
%  this is adequate: the tolerance is wide enough that stochastic SAC
%  exploration reliably crosses the boundary, and the TargetScheduler
%  then advances to the next waypoint, so the agent has no incentive to
%  stay inside. For the 8 mm PICK tolerance, the waypoint is entered
%  early in the episode from a long approach distance with a large
%  number of training episodes, and PickRate = 100 % is achieved. For
%  the 8 mm PLACE tolerance, the agent arrives in Phase 4 from the
%  CRUISE region, ~107 mm away, late in the episode. Along that
%  trajectory there is no local reward signal between d = 107 mm and
%  d = 8 mm: progress reward decays as approach rate slows, and the
%  bonus is zero until d < 8 mm. The deterministic mean policy then
%  converges to ~26 mm — the point at which further approach becomes
%  marginal in progress reward and no bonus is yet available.
%
%  v19.7 — MINIMAL TARGETED FIX
%  -------------------------------------------------------------------------
%  v19.7 keeps the intermediate-waypoint reward of v19.4 unchanged
%  (the 100 % deterministic success rate at LIFT and CRUISE shows that
%  the flat +500/25 mm structure is already well matched to the
%  TargetScheduler threshold). It modifies only the PICK and PLACE
%  bonus, replacing the flat step at d < 8 mm with a linear ramp:
%
%      f(d) = 50 + 500 · (1 − d / 8)      for 0 ≤ d < 8 mm
%
%  giving f(8) = 50 (a small entry bonus that preserves a clear
%  discontinuity at the boundary, matching what the agent already
%  learned in V1), f(4) = 300 and f(0) = 550. The implied gradient
%  inside the tolerance is −500 / 8 = −62.5 /mm, strong enough to pull
%  the policy toward the centre of the tolerance rather than the
%  boundary. No approach zone and no outer ramp are added, so the
%  v19.5 failure mode (reward farming between 25 mm and 80 mm) cannot
%  reappear.
%
%  The clamp, step penalty and asymmetric progress term are untouched.
%  LIFT and CRUISE remain on the v19.4 flat bonus at 25 mm, so the
%  already-stable intermediate behaviour observed across V1 and V1-retry
%  is preserved. Any change in evaluation metrics between V1-retry and
%  this run is therefore attributable to the terminal-waypoint shaping
%  alone.
%
%  PARAMETERS
%  -------------------------------------------------------------------------
%    Step penalty                                : -0.02          (unchanged)
%    Progress coefficient (forward)              : +1000          (unchanged)
%    Progress coefficient (backward)             : +200           (unchanged)
%    Intermediate bonus threshold (LIFT/CRUISE)  :  25 mm         (unchanged)
%    Intermediate bonus amount                   : +500 flat      (unchanged)
%    Terminal bonus threshold (PICK/PLACE)       :   8 mm         (unchanged)
%    Terminal bonus structure                    : graded          (NEW)
%        f(d) = 50 + 500·(1 − d/8)   for d < 8 mm
%        f(8) = 50                   (entry floor)
%        f(0) = 550                  (centre peak)
%        gradient = -62.5 /mm        (interior pull)
%    Reward clamp                                : [-5, +600]     (unchanged)
%
%% =========================================================================

%#codegen

TargetPosition  = TargetPosition(:);
CurrentPosition = CurrentPosition(:);
PLACE           = PlaceTarget(:);
PICK            = PickTarget(:);

persistent prevDist prevTarget

if isempty(prevDist)
    prevDist   = norm(CurrentPosition - TargetPosition) / 1000;
    prevTarget = TargetPosition;
end

if norm(prevTarget - TargetPosition) > 1.0
    prevDist   = norm(CurrentPosition - TargetPosition) / 1000;
    prevTarget = TargetPosition;
end

dist    = norm(CurrentPosition - TargetPosition) / 1000;
dist_mm = dist * 1000;

reward = -0.02;

delta = prevDist - dist;
if delta > 0
    reward = reward + delta * 1000;
else
    reward = reward + delta * 200;
end
prevDist = dist;

isAtPick  = norm(TargetPosition - PICK)  < 1.0;
isAtPlace = norm(TargetPosition - PLACE) < 1.0;

if isAtPick || isAtPlace
    if dist_mm < 8.0
        reward = reward + 50.0 + 500.0 * (1.0 - dist_mm/8.0);
    end
else
    if dist_mm < 25.0
        reward = reward + 500.0;
    end
end

reward = max(-5.0, min(600.0, reward));

end

== matlab function RL_UR3e_Pick_and_Place_Traj/UR3e Pick and Place/Forward Kinematics ==
  data: pos output; theta input
%% =========================================================================
%  FILE        : SolveForwardKinematics.m
%
%  PROJECT     : UR3e Reinforcement Learning Framework
%
%  AUTHOR      : Ahmed Iqdymat
%  DATE        : 18-Mar-2026
%  VERSION     : v5.0  (FINAL)
%
%  AFFILIATION : University Politehnica of Bucharest
%  SUPERVISOR  : Dr. Grigore Stamatescu
%
%  DESCRIPTION
%  -------------------------------------------------------------------------
%  Computes the end-effector Cartesian position of the UR3e robot using
%  standard Denavit–Hartenberg forward kinematics.
%
%  This implementation is designed to be fully compatible with MATLAB
%  code generation and MATLAB Function blocks inside Simulink.
%
%  All DH constants are hardcoded in the function to avoid workspace
%  access or dynamic evaluation.
%
%  CODE GENERATION SAFETY
%  -------------------------------------------------------------------------
%  - No evalin
%  - No assignin
%  - No workspace dependencies
%  - All constants defined locally
%
%  INPUT
%  -------------------------------------------------------------------------
%  theta  : [6x1] joint angles [rad]
%
%  OUTPUT
%  -------------------------------------------------------------------------
%  pos    : [3x1] end-effector position [x;y;z] in millimeters
%
%  CHANGE LOG
%  -------------------------------------------------------------------------
%  v4.0 (09-Mar-2026)
%      Final code-generation safe version for Simulink integration.
%
%% =========================================================================

function pos = SolveForwardKinematics(theta)

%#codegen

%% -------------------------------------------------------------------------
% 1) Input Normalization
% -------------------------------------------------------------------------

theta = theta(:);

%% -------------------------------------------------------------------------
% 2) UR3e DH Parameters
% -------------------------------------------------------------------------
% Format:
% alpha [rad] | a [mm] | d [mm]

alpha = [ pi/2 ;    0   ;    0   ;  pi/2 ; -pi/2 ;   0   ];
a_dh  = [   0  ; -243.55; -213.20;    0  ;    0  ;   0   ];   % mm
d_dh  = [ 151.85;   0   ;    0   ; 131.05;  85.35;  92.10 ];  % mm

%% -------------------------------------------------------------------------
% 3) Forward Kinematics Computation
% -------------------------------------------------------------------------

T = eye(4);

for i = 1:6

    ct = cos(theta(i));
    st = sin(theta(i));

    ca = cos(alpha(i));
    sa = sin(alpha(i));

    ai = a_dh(i);
    di = d_dh(i);

    Ti = [ ct, -st*ca,  st*sa,  ai*ct ;
           st,  ct*ca, -ct*sa,  ai*st ;
            0,     sa,     ca,     di ;
            0,      0,      0,      1 ];

    T = T * Ti;

end

%% -------------------------------------------------------------------------
% 4) Extract End-Effector Position
% -------------------------------------------------------------------------

pos = T(1:3, 4);   % [x; y; z] mm

end

== matlab function RL_UR3e_Pick_and_Place_Traj/UR3e Pick and Place/Observation ==
  data: TargetPosition input; CurrentPosition input; theta input; Omega input; obs output; NextTarget input
function obs = Observation(TargetPosition, CurrentPosition, theta, Omega, NextTarget)
%% =========================================================================
%  Observation v9.0
%  DATE : 08-Apr-2026
%
%  CHANGE FROM v8.0: Added NextTarget direction (24-dim → 27-dim)
%  =========================================================================
%
%  WHY 27-dim:
%  v8.0 gives agent (Target - Current) — direction to CURRENT waypoint.
%  After crossing a waypoint, the agent doesn't know where the NEXT one is.
%  It moves randomly until it stumbles upon it by chance.
%
%  v9.0 adds next_dir = (NextTarget - Current) / 300 — 3 extra dimensions.
%  Now the agent knows WHERE to go after crossing the current waypoint.
%  This converts blind random search into guided navigation.
%
%  STRUCTURE (27-dim):
%  -------------------------------------------------------------------------
%    [1 : 3 ]  pos_near      = (Target - Current) / 100   near-field
%    [4 : 6 ]  pos_far       = (Target - Current) / 300   far-field
%    [7 : 9 ]  next_dir      = (NextTarget - Current) / 300   ← NEW
%    [10:15 ]  sin(theta)
%    [16:21 ]  cos(theta)
%    [22:27 ]  omega_scaled
%
%  INPUTS:
%  TargetPosition  [3x1] mm  — current active waypoint (from TargetScheduler)
%  CurrentPosition [3x1] mm  — EE position (from FK)
%  theta           [6x1] rad — joint angles
%  Omega           [6x1] rad/s — joint velocities
%  NextTarget      [3x1] mm  — next waypoint (from TargetScheduler v3.0) ← NEW
%
%  OUTPUT:
%  obs             [27x1]
%
%% =========================================================================

%#codegen

TargetPosition  = TargetPosition(:);
CurrentPosition = CurrentPosition(:);
theta           = theta(:);
Omega           = Omega(:);
NextTarget      = NextTarget(:);

%% --- Position Error — DUAL SCALE (same as v8.0) ---
error_mm = TargetPosition - CurrentPosition;

pos_near = max(-1, min(1, error_mm / 100));    % near-field [3x1]
pos_far  = max(-1, min(1, error_mm / 300));    % far-field  [3x1]

%% --- Next Target Direction (NEW in v9.0) ---
next_error = NextTarget - CurrentPosition;
next_dir   = max(-1, min(1, next_error / 300)); % far-scale  [3x1]

%% --- Joint Angles ---
theta_sin = sin(theta);   % [6x1]
theta_cos = cos(theta);   % [6x1]

%% --- Joint Velocities ---
omega_scaled      = zeros(6,1);
omega_scaled(1:3) = Omega(1:3) / pi;
omega_scaled(4:6) = Omega(4:6) / (2*pi);
omega_scaled      = max(-1, min(1, omega_scaled));  % [6x1]

%% --- Build Output Vector ---
obs = [ pos_near     ;   %  3  near-field to current target
        pos_far      ;   %  3  far-field to current target
        next_dir     ;   %  3  direction to NEXT target (NEW)
        theta_sin    ;   %  6
        theta_cos    ;   %  6
        omega_scaled ];  %  6
% Total = 27

end

== matlab function RL_UR3e_Pick_and_Place_Traj/UR3e Pick and Place/Done ==
  settings: updateMethod=DISCRETE
  data: TargetPosition input; CurrentPosition input; isdone output; theta input; Omega input; PlaceTarget input
function isdone = Done(TargetPosition, CurrentPosition, theta, Omega, PlaceTarget)
%% =========================================================================
%  Done v8.2 — NP=600 (proven in v19.5)
%  FUNCTION SIGNATURE: UNCHANGED (same 5 inputs as v15.2)
%% =========================================================================

%#codegen

GoalTol_mm      = 5.0;
NoProgressSteps = int32(600);

ThetaMax = 2.0 * pi * ones(6,1);
OmegaMax  = [pi; pi; pi; 2.0*pi; 2.0*pi; 2.0*pi];
VelFactor = 2.0;

PLACE           = PlaceTarget(:);
TargetPosition  = TargetPosition(:);
CurrentPosition = CurrentPosition(:);
theta           = theta(:);
Omega           = Omega(:);

persistent bestDist noProgCount prevTarget

if isempty(bestDist)
    bestDist    = norm(CurrentPosition - TargetPosition);
    noProgCount = int32(0);
    prevTarget  = TargetPosition;
end

if norm(prevTarget - TargetPosition) > 1.0
    bestDist    = norm(CurrentPosition - TargetPosition);
    noProgCount = int32(0);
    prevTarget  = TargetPosition;
end

if any(abs(theta) > ThetaMax)
    isdone = true; return
end

if any(abs(Omega) > OmegaMax * VelFactor)
    isdone = true; return
end

dist_mm = norm(CurrentPosition - TargetPosition);

isAtPlace = norm(TargetPosition - PLACE) < 1.0;
if isAtPlace && dist_mm < GoalTol_mm
    isdone = true; return
end

if dist_mm < GoalTol_mm
    isdone = false; return
end

if dist_mm < bestDist - 1.0
    bestDist    = dist_mm;
    noProgCount = int32(0);
else
    noProgCount = noProgCount + int32(1);
end

isdone = (noProgCount > NoProgressSteps);

end

== matlab function RL_UR3e_Pick_and_Place_Traj/UR3e Pick and Place/Sequential Goal Selector ==
  data: Pick input; Place input; TargetPosition output; CurrentPosition input; phase_out output; dist_out output; NextTarget output
function [TargetPosition, phase_out, dist_out, NextTarget] = TargetScheduler(Pick, Place, CurrentPosition)
%#codegen
%% =========================================================================
%  FILE    : TargetScheduler.m
%  PROJECT : UR3e RL Framework — Project #1 (Clean)
%  VERSION : v4.0
%  DATE    : 21-Apr-2026
%
%  AUTHOR  : Ahmed Iqdymat
%
%  CRITICAL CHANGE FROM v3.1 (v19.9): REMOVED TRANSPORT WAYPOINT
%  -------------------------------------------------------------------------
%  v3.1 (v19.9) used 5 phases:
%     PICK → LIFT → CRUISE → TRANSPORT → PLACE
%  with TRANSPORT = PLACE + [0, 0, +50]  (above PLACE in Z)
%
%  This design created a Z-direction reversal at Phase 4 → 5:
%     Z sequence: 120 → 180 → 265 → 350 → 300
%                                    (↑)   (↓)   ← REVERSAL
%
%  After 4 ascending phases, the policy had encoded "Z+ = reward".
%  The required Z descent for PLACE was fundamentally incompatible
%  with the learned bias. Result: PLACE 0% across all v19.x versions
%  despite TRANSPORT being reached 60-85% of the time.
%
%  v4.0 (Project #1): 4 phases with monotonic Z ascent
%     PICK → LIFT → CRUISE → PLACE
%     Z sequence: 120 → 180 → 265 → 300      (all +Z)
%
%  No Z-reversal. No direction conflict. PLACE is simply the final
%  ascending waypoint, the highest Z target.
%
%  WAYPOINTS
%  -------------------------------------------------------------------------
%    PICK   = [-380, -170, 120]  mm     (grasp target)
%    LIFT   = PICK  + [0, 0, 60]  = [-380, -170, 180]   (Z+60)
%    CRUISE = (LIFT + CRUISE_REF_ANCHOR) mid-height waypoint
%           = [-290, -110, 265]  mm                      (Z+85)
%    PLACE  = [-200,  -50, 300]  mm     (final target)   (Z+35)
%
%  CRUISE position is kept identical to v19.9 because that value was
%  empirically proven to be reachable (100% rate across all v19.5-v19.12
%  runs). Changing CRUISE would require re-learning phases 1-3.
%
%  PER-PHASE TOLERANCES [mm]
%  -------------------------------------------------------------------------
%    Phase 1 PICK   :  8 mm   (grasp precision — terminal target)
%    Phase 2 LIFT   : 25 mm   (transit — lateral of PICK)
%    Phase 3 CRUISE : 25 mm   (transit — mid-height)
%    Phase 4 PLACE  :  8 mm   (release precision — terminal target)
%
%  Final PLACE success (5 mm) is checked in Done.m (not here).
%  This scheduler only determines phase transitions.
%
%  OUTPUTS
%  -------------------------------------------------------------------------
%    TargetPosition [3x1] : current active waypoint to reward against
%    phase_out      [1x1] : current phase number (1..4)
%    dist_out       [1x1] : distance from EE to current target [mm]
%    NextTarget     [3x1] : next waypoint (for Observation v9.0 lookahead)
%
%  INPUTS
%  -------------------------------------------------------------------------
%    Pick            [3x1]  : PICK target from workspace
%    Place           [3x1]  : PLACE target from workspace
%    CurrentPosition [3x1]  : current EE position (from Forward Kinematics)
%
%  LOOKAHEAD (NextTarget) RULES
%  -------------------------------------------------------------------------
%    Phase 1 (PICK)   -> NextTarget = LIFT
%    Phase 2 (LIFT)   -> NextTarget = CRUISE
%    Phase 3 (CRUISE) -> NextTarget = PLACE
%    Phase 4 (PLACE)  -> NextTarget = PLACE  (final, no further lookahead)
%
%% =========================================================================

%% -------------------------------------------------------------------------
% 1) Input normalization
% -------------------------------------------------------------------------
Pick            = Pick(:);
Place           = Place(:);
CurrentPosition = CurrentPosition(:);

%% -------------------------------------------------------------------------
% 2) Waypoint definitions
% -------------------------------------------------------------------------
% NOTE: CRUISE is hardcoded at the proven v19.9 position [-290,-110,265]
%       to preserve learning from v19.5-v19.9 phases 1-3.
%       It is deliberately NOT computed as midpoint of LIFT/PLACE because
%       that midpoint (= [-290,-110,240]) would differ from the value the
%       agent successfully reached in v19.9.

LIFT   = Pick + [0; 0; 60];
CRUISE = [-290; -110; 265];      % v19.9 proven CRUISE (hardcoded for stability)

targets      = zeros(3, 4);
targets(:,1) = Pick;
targets(:,2) = LIFT;
targets(:,3) = CRUISE;
targets(:,4) = Place;

%% -------------------------------------------------------------------------
% 3) Per-phase goal tolerances [mm]
% -------------------------------------------------------------------------
%   Phase 1 PICK   :  8 mm   (precision grasp)
%   Phase 2 LIFT   : 25 mm   (transit)
%   Phase 3 CRUISE : 25 mm   (transit)
%   Phase 4 PLACE  :  8 mm   (precision release)

tols = [8.0; 25.0; 25.0; 8.0];

%% -------------------------------------------------------------------------
% 4) Outputs: preallocate for codegen
% -------------------------------------------------------------------------
TargetPosition = zeros(3,1);
NextTarget     = zeros(3,1);
phase_out      = 1.0;
dist_out       = 0.0;

%% -------------------------------------------------------------------------
% 5) Persistent phase state (cleared by env.ResetFcn at episode start)
% -------------------------------------------------------------------------
persistent phase
if isempty(phase)
    phase = 1.0;
end

%% -------------------------------------------------------------------------
% 6) Phase advancement logic
% -------------------------------------------------------------------------
% Greedy advance: if the agent is inside the tolerance of the current
% waypoint (and possibly subsequent ones in the same frame), advance
% through them. This allows natural overshoot handling.

idx    = max(1, min(4, round(phase)));
target = targets(:, idx);
dist   = norm(CurrentPosition - target);

while phase < 4.0 && dist < tols(idx)
    phase  = phase + 1.0;
    idx    = max(1, min(4, round(phase)));
    target = targets(:, idx);
    dist   = norm(CurrentPosition - target);
end

TargetPosition = target;
phase_out      = phase;
dist_out       = dist;

%% -------------------------------------------------------------------------
% 7) NextTarget (for Observation v9.0 lookahead direction)
% -------------------------------------------------------------------------
nextIdx    = min(4, idx + 1);
NextTarget = targets(:, nextIdx);

end
